simulink model "Satellite_Model_new_seperateSA"  (R2023b)
settings: Solver=ode5  StartTime=0.0  StopTime=10.0  FixedStep=0.1  RelTol=1e-3
undefined symbols (not defined in the file or in its folder): bdf_SA, config_gimbal, epsilon_SA2, f06_SA, gimbal_attach_point, gimbal_cog, gimbal_inertias, gimbal_mass, gimbal_transition_matrix, instrument_attach_point, instrument_inertias, instrument_mass, instrument_transition_matrix, InvDyn, J_B_B, m_B, ObB, ObP1, ObP2, pass, SA, SADM, sig4, unc_freq_SA, uss
libraries: RCTblocks x53, SDTlibV1 x2
(part 1 of 2)
settings Model: Creator=g.iacono  LastModifiedBy=g.iacono

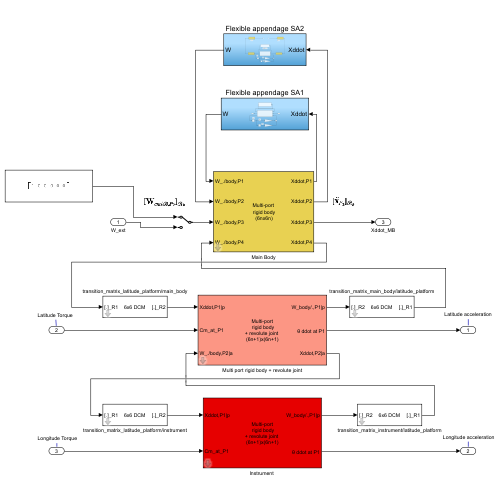
[thumbnail: Simulink's stored preview of the top-level diagram]
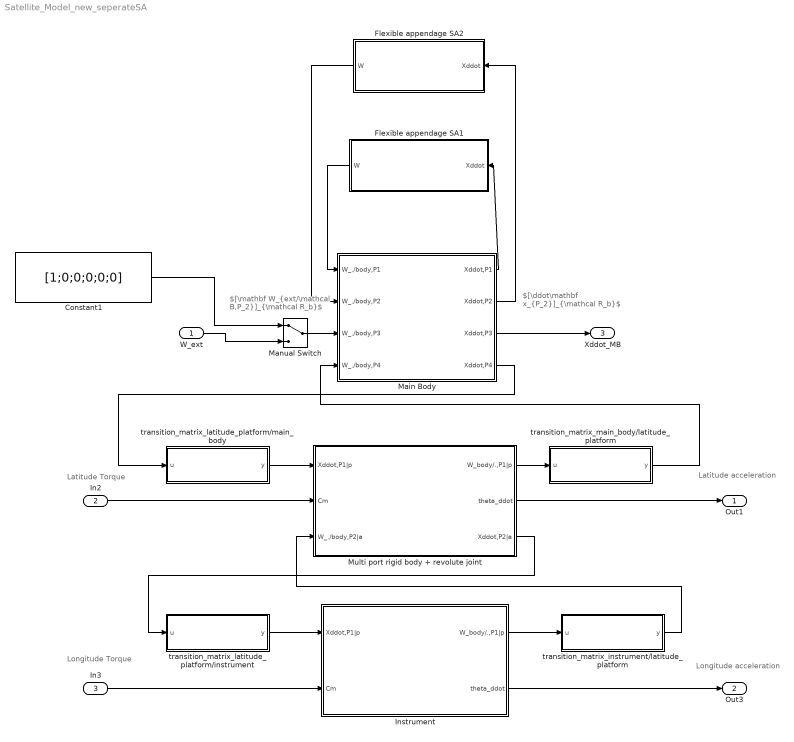
== system Satellite_Model_new_seperateSA ==
  note: Longitude acceleration
  note: Latitude acceleration
  note: $[\ddot\mathbf x_{P_2}]_{\mathcal R_b}$
  note: Longitude Torque
  note: Latitude Torque
  note: $[\mathbf W_{ext/\mathcal B,P_2}]_{\mathcal R_b}$
  W_ext : Inport
  In2 : Inport  Port=2
  In3 : Inport  Port=3
  Constant1 : Constant  Value=[1;0;0;0;0;0]
  Flexible appendage SA1 : Subsystem
  Flexible appendage SA2 : Subsystem
  "Instrument " : Subsystem  mask(Multi-port rigid body with revolute joint (6n+1x6n+1)){m=instrument_mass, Ig=instrument_inertias, OG=instrument_cog-instrument_attach_point, n=1, OP1=[0;0;0], OP2=instrument_attach_point-gimbal_attach_point, OP3=[0;0;0], OP4=[0;0;0], OP5=[0;0;0], ra=[0;1;0], theta=config_gimbal{2}}
      mask prompts: m "Mass (kg)"; Ig "Inertia at G in Ra (kg.m^2)"; OG "OG (3x1 vector in Ra)  (m)"; n "n (number of connection points)"; OP1 "OP1 (3x1 vector in Ra) (m)"; OP2 "OP2 (3x1 vector in Ra) (m)"; OP3 "OP3 (3x1 vector in Ra) (m)"; OP4 "OP4 (3x1 vector in Ra) (m)"; OP5 "OP5 (3x1 vector in Ra) (m)"; ra "ra (joint axis) (3x1 vector)"; theta "Angular configuration (rad)"
      mask help:
      | Computes the (6n+1)x(6n+1) model :
      | - 6x6 transfer from the acceleration twist to the wrench applied by this body to a parent body at port P1 through a revolute joint
      | - the channel # 7 is the transfer:
      |               * from  the  joint torque applied by the input (parent) shaft to the output (body) shaft
      |               * to the relative angular acceleration of the output shaft w.r.t the input shaft.
      | - (n-1) 6x6 transfers from the wrenches applied to this body to the acceleration twists at ports P2,P3,..,
      |
      | Input/Output of port P1 are expressed in the parent frame Rp
      | Input/Output of ports P2,P3,... are expressed in the body frame Ra.
      |
      | O: the body reference point
      | G: the center of mass
      | Pi (i=1:n): the n given connection points or ports (n<6).
      | ra: direction of the revolute joint in the Rp (or Ra)
      | theta: angular configuration of the joint (Ra is obtained from Rp by a rotation of theta around ra).
      |
      | All parameters must be expressed in the body frame Ra.
      | Each parameter can be an uncertain parameter declared with the function ureal (except ra)
      |
      | Rk: if "theta" field is: ureal('NAME',0,'Range',[-pi pi])
      | then, ULINEARIZE will provide a model involving the block named "tan_NAME_div4";
      mask init:
      | MultiPortRigidBodyRev
      mask Help: web('DocMultiportRigidBodyRevolute.html')
      mask TypeOptions n: 1 | 2 | 3 | 4 | 5
      mask DialogControl ParameterGroupVar Prompt: Rigid body parameter
      mask DialogControl port1 Prompt: #1
      mask DialogControl port2 Prompt: #2
      mask DialogControl port3 Prompt: #3
      mask DialogControl port4 Prompt: #4
      mask DialogControl port5 Prompt: #5
      mask DialogControl JointParameters Prompt: Revolute joint parameters
      mask Display:
      | disp('Multi-port\n rigid body\n+ revolute joint \n(6n+1)x(6n+1)')
      | 
      | port_label('input', 1,'Xddot,P1|p')
      | port_label('output',1,'W_body/.,P1|p')
      | port_label('input', 2,'Cm_at_P1')
      | port_label('output',2,'\theta ddot at P1','interpreter','tex')
      | 
      | if n>1
      |     for i=2:n
      |         port_label('input', i+1,['W_./body,P',num2str(i),'|a'])
      |         port_label('output',i+1,['Xddot,P',num2str(i),'|a'])
      |     end
      | end
  Main Body : Subsystem  mask(Multi-port rigid body (6nx6n)){m=m_B, Ig=J_B_B, OG=ObB, n=4, numinv=none, OP1=ObP1, OP2=ObP2, OP3=ObB, OP4=[0;0;0], OP5=[0;0;0]}
      mask prompts: m "Mass (Kg)"; Ig "Inertia (at G, Kg m^2)"; OG "OG (3x1 vector, m)"; n "Number of ports"; numinv "Port to be inverted"; OP1 "OP1 (3x1 vector, m)"; OP2 "OP2 (3x1 vector, m)"; OP3 "OP3 (3x1 vector, m)"; OP4 "OP4 (3x1 vector, m)"; OP5 "OP5 (3x1 vector,m)"
      mask help:
      | 6nx6n dynamic model of a rigid body at n given points (ports) between wrenches applied at the n points (input) and acceleration twists at these points (output).
      |
      | 0: the reference point
      | G: the center of mass
      | Pi (i=1:n): the n given connection points (n<6).
      |
      | All parameters are expressed in the body frame.
      | Each parameter can be an uncertain parameter declared with "ureal"
      |
      | The 6x6 channel associated to one port can be inverted: then the input of this channel is the acceleration twist imposed at this point and the output is the wrench applied by this body.
      mask init:
      | MultiPortRigidBody
      mask Help: web('Docmultiportrigidbody.html')
      mask TypeOptions n: 1 | 2 | 3 | 4 | 5
      mask TypeOptions numinv: none | 1 | 2 | 3 | 4 | 5
      mask DialogControl ParameterGroupVar Prompt: Main parameters
      mask DialogControl port1 Prompt: Port #1
      mask DialogControl port2 Prompt: #2
      mask DialogControl port3 Prompt: #3
      mask DialogControl port4 Prompt: #4
      mask DialogControl port5 Prompt: #5
      mask Display:
      | disp('Multi-port\n rigid body\n (6nx6n)')
      | if n==1,
      |     if numinv-1==1,
      |         port_label('input', 1,'Xddot,P')
      |         port_label('output',1,'W_body/.,P')
      |     else
      |         port_label('input', 1,'W_./body,P')
      |         port_label('output',1,'Xddot,P')
      |     end
      | else
      |     for ii=1:n
      |         if numinv==ii+1,
      |             port_label('output',ii,['W_body/.,P',num2str(ii)])
      |             port_label('input', ii,['Xddot,P',num2str(ii)])
      |         else
      |             port_label('input', ii,['W_./body,P',num2str(ii)])
      |             port_label('output',ii,['Xddot,P',num2str(ii)])
      |         end
      |     end
      | end
  Manual Switch : ManualSwitch
  Multi port rigid body + revolute joint : Subsystem  mask(Multi-port rigid body with revolute joint (6n+1x6n+1)){m=gimbal_mass, Ig=gimbal_inertias, OG=-gimbal_cog+gimbal_attach_point, n=2, OP1=[0;0;0], OP2=-instrument_attach_point+gimbal_attach_point, OP3=[0;0;0], OP4=[0;0;0], OP5=[0;0;0], ra=[1;0;0], theta=config_gimbal{1}}
      mask prompts: m "Mass (kg)"; Ig "Inertia at G in Ra (kg.m^2)"; OG "OG (3x1 vector in Ra)  (m)"; n "n (number of connection points)"; OP1 "OP1 (3x1 vector in Ra) (m)"; OP2 "OP2 (3x1 vector in Ra) (m)"; OP3 "OP3 (3x1 vector in Ra) (m)"; OP4 "OP4 (3x1 vector in Ra) (m)"; OP5 "OP5 (3x1 vector in Ra) (m)"; ra "ra (joint axis) (3x1 vector)"; theta "Angular configuration (rad)"
      mask help:
      | Computes the (6n+1)x(6n+1) model :
      | - 6x6 transfer from the acceleration twist to the wrench applied by this body to a parent body at port P1 through a revolute joint
      | - the channel # 7 is the transfer:
      |               * from  the  joint torque applied by the input (parent) shaft to the output (body) shaft
      |               * to the relative angular acceleration of the output shaft w.r.t the input shaft.
      | - (n-1) 6x6 transfers from the wrenches applied to this body to the acceleration twists at ports P2,P3,..,
      |
      | Input/Output of port P1 are expressed in the parent frame Rp
      | Input/Output of ports P2,P3,... are expressed in the body frame Ra.
      |
      | O: the body reference point
      | G: the center of mass
      | Pi (i=1:n): the n given connection points or ports (n<6).
      | ra: direction of the revolute joint in the Rp (or Ra)
      | theta: angular configuration of the joint (Ra is obtained from Rp by a rotation of theta around ra).
      |
      | All parameters must be expressed in the body frame Ra.
      | Each parameter can be an uncertain parameter declared with the function ureal (except ra)
      |
      | Rk: if "theta" field is: ureal('NAME',0,'Range',[-pi pi])
      | then, ULINEARIZE will provide a model involving the block named "tan_NAME_div4";
      mask init:
      | MultiPortRigidBodyRev
      mask Help: web('DocMultiportRigidBodyRevolute.html')
      mask TypeOptions n: 1 | 2 | 3 | 4 | 5
      mask DialogControl ParameterGroupVar Prompt: Rigid body parameter
      mask DialogControl port1 Prompt: #1
      mask DialogControl port2 Prompt: #2
      mask DialogControl port3 Prompt: #3
      mask DialogControl port4 Prompt: #4
      mask DialogControl port5 Prompt: #5
      mask DialogControl JointParameters Prompt: Revolute joint parameters
      mask Display:
      | disp('Multi-port\n rigid body\n+ revolute joint \n(6n+1)x(6n+1)')
      | 
      | port_label('input', 1,'Xddot,P1|p')
      | port_label('output',1,'W_body/.,P1|p')
      | port_label('input', 2,'Cm_at_P1')
      | port_label('output',2,'\theta ddot at P1','interpreter','tex')
      | 
      | if n>1
      |     for i=2:n
      |         port_label('input', i+1,['W_./body,P',num2str(i),'|a'])
      |         port_label('output',i+1,['Xddot,P',num2str(i),'|a'])
      |     end
      | end
  transition_matrix_instrument/latitude_platform : Subsystem  mask(6x6 Direction cosine matrix (DCM)){rot=instrument_transition_matrix, transp=off}
      mask prompts: rot "3x3 DCM"; transp "Matrix transposed"
      mask help:
      | For 6 d.o.f. body motion (3 translations and 3 rotations), this block Implement the 6x6 rotation matrix (or its transposed) for a given 3x3 DCM.
      |
      | Considering 2 frames R1 and  R2, the DCM between R1 and R2 is defined as the 3x3 matrix where each column is the component vector of each R2 orthogonal unit vector expressed in R1. Thus
      |
      |    [v]_R1 = DCM  * [v]_R2.
      mask init:
      | if transp,
      |     rot=rot';
      | end
      mask Help: web('Doc6dcm.html')
      mask Display:
      | disp('6x6 DCM')
      | if transp
      |     port_label('input', 1, '[.]_R1')
      |     port_label('output', 1, '[.]_R2')
      | else
      |     port_label('input', 1, '[.]_R2')
      |     port_label('output', 1, '[.]_R1')
      | end
  transition_matrix_latitude_platform/instrument : Subsystem  mask(6x6 Direction cosine matrix (DCM)){rot=instrument_transition_matrix, transp=on}
      mask prompts: rot "3x3 DCM"; transp "Matrix transposed"
      mask help:
      | For 6 d.o.f. body motion (3 translations and 3 rotations), this block Implement the 6x6 rotation matrix (or its transposed) for a given 3x3 DCM.
      |
      | Considering 2 frames R1 and  R2, the DCM between R1 and R2 is defined as the 3x3 matrix where each column is the component vector of each R2 orthogonal unit vector expressed in R1. Thus
      |
      |    [v]_R1 = DCM  * [v]_R2.
      mask init:
      | if transp,
      |     rot=rot';
      | end
      mask Help: web('Doc6dcm.html')
      mask Display:
      | disp('6x6 DCM')
      | if transp
      |     port_label('input', 1, '[.]_R1')
      |     port_label('output', 1, '[.]_R2')
      | else
      |     port_label('input', 1, '[.]_R2')
      |     port_label('output', 1, '[.]_R1')
      | end
  transition_matrix_latitude_platform/main_body : Subsystem  mask(6x6 Direction cosine matrix (DCM)){rot=gimbal_transition_matrix, transp=on}
      mask prompts: rot "3x3 DCM"; transp "Matrix transposed"
      mask help:
      | For 6 d.o.f. body motion (3 translations and 3 rotations), this block Implement the 6x6 rotation matrix (or its transposed) for a given 3x3 DCM.
      |
      | Considering 2 frames R1 and  R2, the DCM between R1 and R2 is defined as the 3x3 matrix where each column is the component vector of each R2 orthogonal unit vector expressed in R1. Thus
      |
      |    [v]_R1 = DCM  * [v]_R2.
      mask init:
      | if transp,
      |     rot=rot';
      | end
      mask Help: web('Doc6dcm.html')
      mask Display:
      | disp('6x6 DCM')
      | if transp
      |     port_label('input', 1, '[.]_R1')
      |     port_label('output', 1, '[.]_R2')
      | else
      |     port_label('input', 1, '[.]_R2')
      |     port_label('output', 1, '[.]_R1')
      | end
  transition_matrix_main_body/latitude_platform : Subsystem  mask(6x6 Direction cosine matrix (DCM)){rot=gimbal_transition_matrix, transp=off}
      mask prompts: rot "3x3 DCM"; transp "Matrix transposed"
      mask help:
      | For 6 d.o.f. body motion (3 translations and 3 rotations), this block Implement the 6x6 rotation matrix (or its transposed) for a given 3x3 DCM.
      |
      | Considering 2 frames R1 and  R2, the DCM between R1 and R2 is defined as the 3x3 matrix where each column is the component vector of each R2 orthogonal unit vector expressed in R1. Thus
      |
      |    [v]_R1 = DCM  * [v]_R2.
      mask init:
      | if transp,
      |     rot=rot';
      | end
      mask Help: web('Doc6dcm.html')
      mask Display:
      | disp('6x6 DCM')
      | if transp
      |     port_label('input', 1, '[.]_R1')
      |     port_label('output', 1, '[.]_R2')
      | else
      |     port_label('input', 1, '[.]_R2')
      |     port_label('output', 1, '[.]_R1')
      | end
  Out1 : Outport  VectorParamsAs1DForOutWhenUnconnected=off
  Out3 : Outport  Port=2  VectorParamsAs1DForOutWhenUnconnected=off
  Xddot_MB : Outport  Port=3
  wires:
  Multi port rigid body + revolute joint/3(Xddot,P2|a) -> transition_matrix_latitude_platform/instrument/1(u)
  Main Body/3(Xddot,P3) -> Xddot_MB/1
  W_ext/1 -> Manual Switch/2
  "Instrument "/2(theta_ddot) -> Out3/1
  In3/1 -> "Instrument "/2(Cm)
  transition_matrix_latitude_platform/instrument/1(y) -> "Instrument "/1(Xddot,P1|p)
  Multi port rigid body + revolute joint/2(theta_ddot) -> Out1/1
  transition_matrix_latitude_platform/main_body/1(y) -> Multi port rigid body + revolute joint/1(Xddot,P1|p)
  Multi port rigid body + revolute joint/1(W_body/.,P1|p) -> transition_matrix_main_body/latitude_platform/1(u)
  "Instrument "/1(W_body/.,P1|p) -> transition_matrix_instrument/latitude_platform/1(u)
  Flexible appendage SA1/1(W) -> Main Body/1(W_./body,P1)
  transition_matrix_main_body/latitude_platform/1(y) -> Main Body/4(W_./body,P4)
  transition_matrix_instrument/latitude_platform/1(y) -> Multi port rigid body + revolute joint/3(W_./body,P2|a)
  In2/1 -> Multi port rigid body + revolute joint/2(Cm)
  Main Body/1(Xddot,P1) -> Flexible appendage SA1/1(Xddot)
  Main Body/4(Xddot,P4) -> transition_matrix_latitude_platform/main_body/1(u)
  Main Body/2(Xddot,P2) -> Flexible appendage SA2/1(Xddot)
  Flexible appendage SA2/1(W) -> Main Body/2(W_./body,P2)
  Manual Switch/1 -> Main Body/3(W_./body,P3)
  Constant1/1 -> Manual Switch/1

== system Satellite_Model_new_seperateSA/Flexible appendage SA1 ==
  note: $\dot{\delta\theta}_1$
  note: $\delta\theta_1$
  note: $\ddot{\delta\theta}_1$
  Xddot : Inport
  Gain1 : Gain  Gain=SADM.damping
  Gain4 : Gain  Gain=SADM.Stiffness
  Integrator1 : Integrator
  Integrator4 : Integrator
  SADM1 : SDTlibV1/6 dof mechanisms/Revolute joint + configuration  ra=[1;0;0]  Jr=1e-9  theta=theta_SA
      settings: SourceProductName=SDTlib
  Solar Array 1 : Subsystem  mask(NINOP Model of a Nastran body){fbdf=bdf_SA, ff06=f06_SA, P_gp=SA.pointP, C_gp=[], nf=SA.n_modes, Xi=SA.damping_ratio, uw_var=unc_freq_SA, Nflex_w=SA.n_unc, uls_var=SA.MPCunc, Nflex_LP=SA.n_MPCunc, uev_var=0, Nflex_EV=0}
      mask prompts: fbdf "Name of the .bdf file (without extension)"; ff06 "Name of the .f06 file (without extension)"; P_gp "Node number corresponding to the point P (connection with parent body)"; C_gp "Node numbers corresponding to the points C (connections with child bodies)"; nf "Number of modes to be considered"; Xi "Common damping ratio"; uw_var "uncertainties (%)"; Nflex_w "number of flexible modes (integer)"; uls_var "uncertainties (%)"; Nflex_LP "number of flexible modes (integer)"; uev_var "uncertainties (%)"; Nflex_EV "number of flexible modes (integer)"
      mask help:
      | NINOP 6(n+1)x6(n+1) model of a flexible body at points C (connection point with the child  bodies) and point P (connection point with a parent body).
      | * 6nx6n transfer between the wrench applied to this body at the child points C  and accelaretion twist at these points
      | * 6x6 transfer between the acceleration twist at the "parent" point P  and the wrench applied by this body at this point
      | The model is expressed In the (inherit) body frame.
      |
      | Model is built from  the data provided by Patran/Nastran analysis output files.
      | Uncertainties can be added to the main parameters
      mask init:
      | n = length(C_gp);
      | NastranBodyNPort
      mask Help: web('DocNPortNastranBody.html')
      mask DialogControl Container2 Prompt: Main parameters
      mask DialogControl Container6 Prompt: Parametric uncertainties:
      mask DialogControl Container8 Prompt: Frequencies
      mask DialogControl Control18 Prompt: A common relative uncertainty (%) on the first flexible mode frequencies can be added (uncertainties can be changed later)
      mask DialogControl Control3 Prompt: The uncertain frequency is named: 'w_name_i' where:
      mask DialogControl Control4 Prompt: * 'name' is the current block name (reduced to its alphanumeric characters).
      mask DialogControl Control17 Prompt: * 'i' is the flexible mode number (increasing frequency order)
      mask DialogControl Container9 Prompt: Modal participation factors
      mask DialogControl Control20 Prompt: A common relative uncertainty (%) on the modal participation factors of the first flexible modes can be added (uncertainties can be changed later)
      mask DialogControl Control6 Prompt: The uncertain modal participation factor is named: 'LP_name_iXX' where:
      mask DialogControl Control7 Prompt: *  'name' is the current block name (reduced to its alphanumeric characters),
      mask DialogControl Control8 Prompt: * 'i' is the flexible mode number (increasing frequency order),
      mask DialogControl Control9 Prompt: * 'XX' = 'Tx', 'Ty', 'Tz', 'Rx', 'Ry', 'Rz'.
      mask DialogControl Container10 Prompt: Modal shapes
      mask DialogControl Control21 Prompt: A common relative uncertainty (%) on each eigen vector components at points C for the first flexible modes can be added (uncertainties can be changed later)
      mask DialogControl Control16 Prompt: WARNING: can generate very long process time !!
      mask DialogControl Control11 Prompt: The uncertain component is named: "EV_name_Cj_iXX' where:
      mask DialogControl Control12 Prompt: * 'name' is the current block name (reduced to its alphanumeric characters).
      mask DialogControl Control13 Prompt: * 'j' is the point C number,
      mask DialogControl Control14 Prompt: * 'i' is the flexible mode number (increasing frequency order),
      mask DialogControl Control15 Prompt: * 'XX' = 'Tx', 'Ty', 'Tz', 'Rx', 'Ry', 'Rz'.
      mask Display:
      | disp('NINOP\n Nastran body\n (6(n+1)x6(n+1))')
      | 
      | 
      | for ii=1:n
      |         port_label('input', ii,['W_./body,C',num2str(ii)])
      |         port_label('output',ii,['Xddot,C',num2str(ii)])
      | end
      | 
      | port_label('input', n+1,'Xddot,P')
      | port_label('output',n+1,'Wbody/.,P')
  Sum4 : Sum  Inputs=++|
  W : Outport
  wires:
  SADM1/2 -> W/1
  Xddot/1 -> SADM1/2
  Sum4/1 -> SADM1/3
  Integrator1/1 -> Integrator4/1, Gain1/1
  Gain1/1 -> Sum4/1
  Integrator4/1 -> Gain4/1
  Gain4/1 -> Sum4/2
  SADM1/3 -> Integrator1/1
  SADM1/1 -> Solar Array 1/1(Xddot,P)
  Solar Array 1/1(W_body/.,P) -> SADM1/1

== system Satellite_Model_new_seperateSA/Flexible appendage SA2 ==
  note: $-[\mathbf M^{\mathcal A_2}_{P_2}]_{\mathcal R_{a_2}}(\mathrm s)$
  note: $\mathbf P_{a_2(0)/b}$
  note: $\mathbf P_{a_2(0)/b}^T$
  note: $\ddot{\delta\theta}_2$
  note: $\delta\theta_2$
  note: $\dot{\delta\theta}_2$
  Xddot : Inport
  6x6 DCM1 : Subsystem  mask(6x6 Direction cosine matrix (DCM)){rot=[-1 0 0;0 -1 0;0 0 1], transp=off}
      mask prompts: rot "3x3 DCM"; transp "Matrix transposed"
      mask help:
      | For 6 d.o.f. body motion (3 translations and 3 rotations), this block Implement the 6x6 rotation matrix (or its transposed) for a given 3x3 DCM.
      |
      | Considering 2 frames R1 and  R2, the DCM between R1 and R2 is defined as the 3x3 matrix where each column is the component vector of each R2 orthogonal unit vector expressed in R1. Thus
      |
      |    [v]_R1 = DCM  * [v]_R2.
      mask init:
      | if transp,
      |     rot=rot';
      | end
      mask Help: web('Doc6dcm.html')
      mask Display:
      | disp('6x6 DCM')
      | if transp
      |     port_label('input', 1, '[.]_R1')
      |     port_label('output', 1, '[.]_R2')
      | else
      |     port_label('input', 1, '[.]_R2')
      |     port_label('output', 1, '[.]_R1')
      | end
  6x6 DCM2 : Subsystem  mask(6x6 Direction cosine matrix (DCM)){rot=[-1 0 0;0 -1 0;0 0 1], transp=on}
      mask prompts: rot "3x3 DCM"; transp "Matrix transposed"
      mask help:
      | For 6 d.o.f. body motion (3 translations and 3 rotations), this block Implement the 6x6 rotation matrix (or its transposed) for a given 3x3 DCM.
      |
      | Considering 2 frames R1 and  R2, the DCM between R1 and R2 is defined as the 3x3 matrix where each column is the component vector of each R2 orthogonal unit vector expressed in R1. Thus
      |
      |    [v]_R1 = DCM  * [v]_R2.
      mask init:
      | if transp,
      |     rot=rot';
      | end
      mask Help: web('Doc6dcm.html')
      mask Display:
      | disp('6x6 DCM')
      | if transp
      |     port_label('input', 1, '[.]_R1')
      |     port_label('output', 1, '[.]_R2')
      | else
      |     port_label('input', 1, '[.]_R2')
      |     port_label('output', 1, '[.]_R1')
      | end
  6x6 v-u_rotation2 : Subsystem  mask(6x6 rotation matrix (around a given axis)){ra=[-1;0;0], theta=epsilon_SA2, transp=on}
      mask prompts: ra "Rotation axis (3x1 vector)"; theta "Angle (rad)"; transp "Matrix transposed"
      mask help:
      | For 6 d.o.f. body motion (3 translations and 3 rotations), this block Implement the 6x6 rotation matrix (or its transposed) for a given angle around a given axis.
      |
      | Angle  (rad) can be an uncertain parameter declared with "ureal" with mode 'Range'
      | Ex: ureal('NAME',0,'Range',[-pi pi])
      | Then, ULINEARIZE will provide a model involving the block named "tan_NAME_div4".
      mask init:
      | vUrotation3x3
      mask Help: web('Doc6vurotation.html')
      mask Display:
      | disp('v-rot\n6x6')
      | if transp
      |     port_label('input', 1, '[.]_R1')
      |     port_label('output', 1, '[.]_R2')
      | else
      |     port_label('input', 1, '[.]_R2')
      |     port_label('output', 1, '[.]_R1')
      | end
  6x6 v-u_rotation3 : Subsystem  mask(6x6 rotation matrix (around a given axis)){ra=[-1;0;0], theta=epsilon_SA2, transp=off}
      mask prompts: ra "Rotation axis (3x1 vector)"; theta "Angle (rad)"; transp "Matrix transposed"
      mask help:
      | For 6 d.o.f. body motion (3 translations and 3 rotations), this block Implement the 6x6 rotation matrix (or its transposed) for a given angle around a given axis.
      |
      | Angle  (rad) can be an uncertain parameter declared with "ureal" with mode 'Range'
      | Ex: ureal('NAME',0,'Range',[-pi pi])
      | Then, ULINEARIZE will provide a model involving the block named "tan_NAME_div4".
      mask init:
      | vUrotation3x3
      mask Help: web('Doc6vurotation.html')
      mask Display:
      | disp('v-rot\n6x6')
      | if transp
      |     port_label('input', 1, '[.]_R1')
      |     port_label('output', 1, '[.]_R2')
      | else
      |     port_label('input', 1, '[.]_R2')
      |     port_label('output', 1, '[.]_R1')
      | end
  Gain2 : Gain  Gain=SADM.damping
  Gain3 : Gain  Gain=SADM.Stiffness
  Integrator2 : Integrator
  Integrator3 : Integrator
  SADM2 : SDTlibV1/6 dof mechanisms/Revolute joint + configuration  ra=[-1;0;0]  Jr=1e-9  theta=theta_SA
      settings: SourceProductName=SDTlib
  Solar Array 2 : Subsystem  mask(NINOP Model of a Nastran body){fbdf=bdf_SA, ff06=f06_SA, P_gp=SA.pointP, C_gp=[], nf=SA.n_modes, Xi=SA.damping_ratio, uw_var=unc_freq_SA, Nflex_w=SA.n_unc, uls_var=SA.MPCunc, Nflex_LP=SA.n_MPCunc, uev_var=0, Nflex_EV=0}
      mask prompts: fbdf "Name of the .bdf file (without extension)"; ff06 "Name of the .f06 file (without extension)"; P_gp "Node number corresponding to the point P (connection with parent body)"; C_gp "Node numbers corresponding to the points C (connections with child bodies)"; nf "Number of modes to be considered"; Xi "Common damping ratio"; uw_var "uncertainties (%)"; Nflex_w "number of flexible modes (integer)"; uls_var "uncertainties (%)"; Nflex_LP "number of flexible modes (integer)"; uev_var "uncertainties (%)"; Nflex_EV "number of flexible modes (integer)"
      mask help:
      | NINOP 6(n+1)x6(n+1) model of a flexible body at points C (connection point with the child  bodies) and point P (connection point with a parent body).
      | * 6nx6n transfer between the wrench applied to this body at the child points C  and accelaretion twist at these points
      | * 6x6 transfer between the acceleration twist at the "parent" point P  and the wrench applied by this body at this point
      | The model is expressed In the (inherit) body frame.
      |
      | Model is built from  the data provided by Patran/Nastran analysis output files.
      | Uncertainties can be added to the main parameters
      mask init:
      | n = length(C_gp);
      | NastranBodyNPort
      mask Help: web('DocNPortNastranBody.html')
      mask DialogControl Container2 Prompt: Main parameters
      mask DialogControl Container6 Prompt: Parametric uncertainties:
      mask DialogControl Container8 Prompt: Frequencies
      mask DialogControl Control18 Prompt: A common relative uncertainty (%) on the first flexible mode frequencies can be added (uncertainties can be changed later)
      mask DialogControl Control3 Prompt: The uncertain frequency is named: 'w_name_i' where:
      mask DialogControl Control4 Prompt: * 'name' is the current block name (reduced to its alphanumeric characters).
      mask DialogControl Control17 Prompt: * 'i' is the flexible mode number (increasing frequency order)
      mask DialogControl Container9 Prompt: Modal participation factors
      mask DialogControl Control20 Prompt: A common relative uncertainty (%) on the modal participation factors of the first flexible modes can be added (uncertainties can be changed later)
      mask DialogControl Control6 Prompt: The uncertain modal participation factor is named: 'LP_name_iXX' where:
      mask DialogControl Control7 Prompt: *  'name' is the current block name (reduced to its alphanumeric characters),
      mask DialogControl Control8 Prompt: * 'i' is the flexible mode number (increasing frequency order),
      mask DialogControl Control9 Prompt: * 'XX' = 'Tx', 'Ty', 'Tz', 'Rx', 'Ry', 'Rz'.
      mask DialogControl Container10 Prompt: Modal shapes
      mask DialogControl Control21 Prompt: A common relative uncertainty (%) on each eigen vector components at points C for the first flexible modes can be added (uncertainties can be changed later)
      mask DialogControl Control16 Prompt: WARNING: can generate very long process time !!
      mask DialogControl Control11 Prompt: The uncertain component is named: "EV_name_Cj_iXX' where:
      mask DialogControl Control12 Prompt: * 'name' is the current block name (reduced to its alphanumeric characters).
      mask DialogControl Control13 Prompt: * 'j' is the point C number,
      mask DialogControl Control14 Prompt: * 'i' is the flexible mode number (increasing frequency order),
      mask DialogControl Control15 Prompt: * 'XX' = 'Tx', 'Ty', 'Tz', 'Rx', 'Ry', 'Rz'.
      mask Display:
      | disp('NINOP\n Nastran body\n (6(n+1)x6(n+1))')
      | 
      | 
      | for ii=1:n
      |         port_label('input', ii,['W_./body,C',num2str(ii)])
      |         port_label('output',ii,['Xddot,C',num2str(ii)])
      | end
      | 
      | port_label('input', n+1,'Xddot,P')
      | port_label('output',n+1,'Wbody/.,P')
  Sum3 : Sum  Inputs=++|
  W : Outport
  wires:
  SADM2/1 -> Solar Array 2/1(Xddot,P)
  Xddot/1 -> 6x6 DCM2/1(u)
  6x6 DCM1/1(y) -> W/1
  6x6 DCM2/1(y) -> 6x6 v-u_rotation2/1(u)
  Solar Array 2/1(W_body/.,P) -> SADM2/1
  SADM2/2 -> 6x6 v-u_rotation3/1(u)
  6x6 v-u_rotation2/1(y) -> SADM2/2
  6x6 v-u_rotation3/1(y) -> 6x6 DCM1/1(u)
  SADM2/3 -> Integrator2/1
  Gain3/1 -> Sum3/2
  Integrator3/1 -> Gain3/1
  Gain2/1 -> Sum3/1
  Integrator2/1 -> Integrator3/1, Gain2/1
  Sum3/1 -> SADM2/3

== system Satellite_Model_new_seperateSA/Instrument  ==
  Xddot,P1|p : Inport
  Cm : Inport  Port=2
  Multi port rigid body : Subsystem  mask(Multi-port rigid body (6nx6n)){m=instrument_mass, Ig=[1 0 0;0 0.0005 0;0 0 0.001], OG=instrument_cog-instrument_attach_point, n=1, numinv=1, OP1=[0;0;0], OP2=instrument_attach_point-gimbal_attach_point, OP3=[0;0;0], OP4=[0;0;0], OP5=[0;0;0]}
      mask prompts: m "Mass (Kg)"; Ig "Inertia (at G, Kg m^2)"; OG "OG (3x1 vector, m)"; n "Number of ports"; numinv "Port to be inverted"; OP1 "OP1 (3x1 vector, m)"; OP2 "OP2 (3x1 vector, m)"; OP3 "OP3 (3x1 vector, m)"; OP4 "OP4 (3x1 vector, m)"; OP5 "OP5 (3x1 vector,m)"
      mask help:
      | 6nx6n inverse dynamic model between:
      |    *  wrenches applied to this body at the given n points,
      |    * acceleration twiists at he n given points.
      |
      | The 6x6 channel asociated to a single given point can be inverted
      mask init:
      | MultiPortRigidBody
      mask Help: web('Docmultiportrigidbody.html')
      mask TypeOptions n: 1 | 2 | 3 | 4 | 5
      mask TypeOptions numinv: none | 1 | 2 | 3 | 4 | 5
      mask DialogControl Control1 Prompt: Inverse Dynamic model of a rigid body at n given points (ports):
      mask DialogControl Control2 Prompt: 6nx6n transfer between wrenches applied at the n points and accelaretion twists at these points
      mask DialogControl Control3 Prompt: 0: the reference point
      mask DialogControl Control4 Prompt: G: the center of mass
      mask DialogControl Control5 Prompt: Pi (i=1:n): the n given connection points (n<6).
      mask DialogControl Control6 Prompt: All parameters are expressed in the body frame.
      mask DialogControl Control7 Prompt: Each parameter can be an uncertain parameter declared with "ureal"
      mask DialogControl Control8 Prompt: The 6x6 channel associated to one port can be inverted: then the input of this channel is the acceleration twist imposed at this point and the output is the wrench applied by this body.
      mask DialogControl ParameterGroupVar Prompt: Main parameters
      mask DialogControl port1 Prompt: Port #1
      mask DialogControl port2 Prompt: #2
      mask DialogControl port3 Prompt: #3
      mask DialogControl port4 Prompt: #4
      mask DialogControl port5 Prompt: #5
      mask Display:
      | disp('Multi-port\n rigid body\n (6nx6n)')
      | if n==1,
      |     if numinv-1==1,
      |         port_label('input', 1,'Xddot,P')
      |         port_label('output',1,'W_body/.,P')
      |     else
      |         port_label('input', 1,'W_./body,P')
      |         port_label('output',1,'Xddot,P')
      |     end
      | else
      |     for ii=1:n
      |         if numinv==ii+1,
      |             port_label('output',ii,['W_body/.,P',num2str(ii)])
      |             port_label('input', ii,['Xddot,P',num2str(ii)])
      |         else
      |             port_label('input', ii,['W_./body,P',num2str(ii)])
      |             port_label('output',ii,['Xddot,P',num2str(ii)])
      |         end
      |     end
      | end
  Revolute joint + configuration : Subsystem  mask(Revolute joint){ra=[0;1;0], Jr=0.0005, theta=config_gimbal{2}}
      mask prompts: ra "Direction of the joint in the load frame (3x1 vector)"; Jr "Rotor inertia (kg.m^2)"; theta "Angular configuration (rad)"
      mask help:
      | This block implement the TITOP model of of a revolute joint.
      | The last channel is the transfer between the torque applied inside the joint by the input shaft to the output shaft and the relative angular acceleration of the output shaft w.r.t the input shaft.
      |
      | Angular configuration can be a vayring parameter: Ex:
      | ureal('NAME',0,'Range',[-pi pi])
      |
      | Then, ULINEARIZE will provide a model involving the block named "tan_NAME_div4";
      mask init:
      | pass=ra2DCMi(ra);
      mask Help: web('DocRevoluteJoint_configuration.html')
      mask Display:
      | disp('Revolute joint\nTITOP model\n+ angle configuration')
      | port_label('input', 1, 'W_./r|a')
      | port_label('output', 1, 'Xddot_out|a')
      | port_label('input', 2, 'Xddot_in|p')
      | port_label('output', 2, 'W_r/.|p')
      | port_label('input', 3, 'Cm')
      | port_label('output', 3, '\theta ddot','interpreter','tex')
  W_body/.,P1|p : Outport  VectorParamsAs1DForOutWhenUnconnected=off
  theta_ddot : Outport  Port=2  VectorParamsAs1DForOutWhenUnconnected=off
  wires:
  Revolute joint + configuration/1(Xddot_out|a) -> Multi port rigid body/1(Xddot,P1)
  Multi port rigid body/1(W_body/.,P1) -> Revolute joint + configuration/1(W_./r|a)
  Xddot,P1|p/1 -> Revolute joint + configuration/2(Xddot_in|p)
  Cm/1 -> Revolute joint + configuration/3(Cm)
  Revolute joint + configuration/2(W_r/.|p) -> W_body/.,P1|p/1
  Revolute joint + configuration/3(Theta_ddot) -> theta_ddot/1

== system Satellite_Model_new_seperateSA/Main Body ==
  W_./body,P1 : Inport  PortDimensions=6
  W_./body,P2 : Inport  Port=2  PortDimensions=6
  W_./body,P3 : Inport  Port=3  PortDimensions=6
  W_./body,P4 : Inport  Port=4  PortDimensions=6
  Demux : Demux  Outputs=[6 6 6 6]
  Gain : RCTblocks/Uncertain State Space  Tag=USS  USystem=uss(InvDyn)  UValue=[]  X0=[]  uX0=[]
  Mux : Mux  Inputs=[6 6 6 6]
  Xddot,P1 : Outport
  Xddot,P2 : Outport  Port=2
  Xddot,P3 : Outport  Port=3
  Xddot,P4 : Outport  Port=4
  wires:
  Mux/1 -> Gain/1
  Gain/1 -> Demux/1
  W_./body,P1/1 -> Mux/1
  Demux/1 -> Xddot,P1/1
  W_./body,P2/1 -> Mux/2
  Demux/2 -> Xddot,P2/1
  W_./body,P3/1 -> Mux/3
  Demux/3 -> Xddot,P3/1
  W_./body,P4/1 -> Mux/4
  Demux/4 -> Xddot,P4/1

== system Satellite_Model_new_seperateSA/Multi port rigid body + revolute joint ==
  Xddot,P1|p : Inport
  Cm : Inport  Port=2
  W_./body,P2|a : Inport  Port=3
  Multi port rigid body : Subsystem  mask(Multi-port rigid body (6nx6n)){m=gimbal_mass, Ig=[-3.1995 0 0;0 4 0;0 0 0.001], OG=-gimbal_cog+gimbal_attach_point, n=2, numinv=1, OP1=[0;0;0], OP2=-instrument_attach_point+gimbal_attach_point, OP3=[0;0;0], OP4=[0;0;0], OP5=[0;0;0]}
      mask prompts: m "Mass (Kg)"; Ig "Inertia (at G, Kg m^2)"; OG "OG (3x1 vector, m)"; n "Number of ports"; numinv "Port to be inverted"; OP1 "OP1 (3x1 vector, m)"; OP2 "OP2 (3x1 vector, m)"; OP3 "OP3 (3x1 vector, m)"; OP4 "OP4 (3x1 vector, m)"; OP5 "OP5 (3x1 vector,m)"
      mask help:
      | 6nx6n inverse dynamic model between:
      |    *  wrenches applied to this body at the given n points,
      |    * acceleration twiists at he n given points.
      |
      | The 6x6 channel asociated to a single given point can be inverted
      mask init:
      | MultiPortRigidBody
      mask Help: web('Docmultiportrigidbody.html')
      mask TypeOptions n: 1 | 2 | 3 | 4 | 5
      mask TypeOptions numinv: none | 1 | 2 | 3 | 4 | 5
      mask DialogControl Control1 Prompt: Inverse Dynamic model of a rigid body at n given points (ports):
      mask DialogControl Control2 Prompt: 6nx6n transfer between wrenches applied at the n points and accelaretion twists at these points
      mask DialogControl Control3 Prompt: 0: the reference point
      mask DialogControl Control4 Prompt: G: the center of mass
      mask DialogControl Control5 Prompt: Pi (i=1:n): the n given connection points (n<6).
      mask DialogControl Control6 Prompt: All parameters are expressed in the body frame.
      mask DialogControl Control7 Prompt: Each parameter can be an uncertain parameter declared with "ureal"
      mask DialogControl Control8 Prompt: The 6x6 channel associated to one port can be inverted: then the input of this channel is the acceleration twist imposed at this point and the output is the wrench applied by this body.
      mask DialogControl ParameterGroupVar Prompt: Main parameters
      mask DialogControl port1 Prompt: Port #1
      mask DialogControl port2 Prompt: #2
      mask DialogControl port3 Prompt: #3
      mask DialogControl port4 Prompt: #4
      mask DialogControl port5 Prompt: #5
      mask Display:
      | disp('Multi-port\n rigid body\n (6nx6n)')
      | if n==1,
      |     if numinv-1==1,
      |         port_label('input', 1,'Xddot,P')
      |         port_label('output',1,'W_body/.,P')
      |     else
      |         port_label('input', 1,'W_./body,P')
      |         port_label('output',1,'Xddot,P')
      |     end
      | else
      |     for ii=1:n
      |         if numinv==ii+1,
      |             port_label('output',ii,['W_body/.,P',num2str(ii)])
      |             port_label('input', ii,['Xddot,P',num2str(ii)])
      |         else
      |             port_label('input', ii,['W_./body,P',num2str(ii)])
      |             port_label('output',ii,['Xddot,P',num2str(ii)])
      |         end
      |     end
      | end
  Revolute joint + configuration : Subsystem  mask(Revolute joint){ra=[1;0;0], Jr=3.2005, theta=config_gimbal{1}}
      mask prompts: ra "Direction of the joint in the load frame (3x1 vector)"; Jr "Rotor inertia (kg.m^2)"; theta "Angular configuration (rad)"
      mask help:
      | This block implement the TITOP model of of a revolute joint.
      | The last channel is the transfer between the torque applied inside the joint by the input shaft to the output shaft and the relative angular acceleration of the output shaft w.r.t the input shaft.
      |
      | Angular configuration can be a vayring parameter: Ex:
      | ureal('NAME',0,'Range',[-pi pi])
      |
      | Then, ULINEARIZE will provide a model involving the block named "tan_NAME_div4";
      mask init:
      | pass=ra2DCMi(ra);
      mask Help: web('DocRevoluteJoint_configuration.html')
      mask Display:
      | disp('Revolute joint\nTITOP model\n+ angle configuration')
      | port_label('input', 1, 'W_./r|a')
      | port_label('output', 1, 'Xddot_out|a')
      | port_label('input', 2, 'Xddot_in|p')
      | port_label('output', 2, 'W_r/.|p')
      | port_label('input', 3, 'Cm')
      | port_label('output', 3, '\theta ddot','interpreter','tex')
  W_body/.,P1|p : Outport  VectorParamsAs1DForOutWhenUnconnected=off
  theta_ddot : Outport  Port=2  VectorParamsAs1DForOutWhenUnconnected=off
  Xddot,P2|a : Outport  Port=3
  wires:
  Revolute joint + configuration/1(Xddot_out|a) -> Multi port rigid body/1(Xddot,P1)
  Multi port rigid body/1(W_body/.,P1) -> Revolute joint + configuration/1(W_./r|a)
  Xddot,P1|p/1 -> Revolute joint + configuration/2(Xddot_in|p)
  Cm/1 -> Revolute joint + configuration/3(Cm)
  Revolute joint + configuration/2(W_r/.|p) -> W_body/.,P1|p/1
  Revolute joint + configuration/3(Theta_ddot) -> theta_ddot/1
  W_./body,P2|a/1 -> Multi port rigid body/2(W_./body,P2)
  Multi port rigid body/2(Xddot,P2) -> Xddot,P2|a/1

== system Satellite_Model_new_seperateSA/transition_matrix_instrument//latitude_platform ==
  u : Inport  PortDimensions=6
  Demux : Demux  Outputs=[3 3]
  Mux : Mux  Inputs=[3 3]
  rotation : Gain  Gain=rot  Multiplication=Matrix(K*u) (u vector)
  translation : Gain  Gain=rot  Multiplication=Matrix(K*u) (u vector)
  y : Outport  VectorParamsAs1DForOutWhenUnconnected=off
  wires:
  rotation/1 -> Mux/2
  translation/1 -> Mux/1
  Demux/1 -> translation/1
  u/1 -> Demux/1
  Mux/1 -> y/1
  Demux/2 -> rotation/1

== system Satellite_Model_new_seperateSA/transition_matrix_latitude_platform//instrument ==
  u : Inport  PortDimensions=6
  Demux : Demux  Outputs=[3 3]
  Mux : Mux  Inputs=[3 3]
  rotation : Gain  Gain=rot  Multiplication=Matrix(K*u) (u vector)
  translation : Gain  Gain=rot  Multiplication=Matrix(K*u) (u vector)
  y : Outport  VectorParamsAs1DForOutWhenUnconnected=off
  wires:
  Demux/2 -> rotation/1
  Mux/1 -> y/1
  u/1 -> Demux/1
  Demux/1 -> translation/1
  translation/1 -> Mux/1
  rotation/1 -> Mux/2

== system Satellite_Model_new_seperateSA/transition_matrix_latitude_platform//main_body ==
  u : Inport  PortDimensions=6
  Demux : Demux  Outputs=[3 3]
  Mux : Mux  Inputs=[3 3]
  rotation : Gain  Gain=rot  Multiplication=Matrix(K*u) (u vector)
  translation : Gain  Gain=rot  Multiplication=Matrix(K*u) (u vector)
  y : Outport  VectorParamsAs1DForOutWhenUnconnected=off
  wires:
  rotation/1 -> Mux/2
  translation/1 -> Mux/1
  Demux/1 -> translation/1
  u/1 -> Demux/1
  Mux/1 -> y/1
  Demux/2 -> rotation/1

== system Satellite_Model_new_seperateSA/transition_matrix_main_body//latitude_platform ==
  u : Inport  PortDimensions=6
  Demux : Demux  Outputs=[3 3]
  Mux : Mux  Inputs=[3 3]
  rotation : Gain  Gain=rot  Multiplication=Matrix(K*u) (u vector)
  translation : Gain  Gain=rot  Multiplication=Matrix(K*u) (u vector)
  y : Outport  VectorParamsAs1DForOutWhenUnconnected=off
  wires:
  rotation/1 -> Mux/2
  translation/1 -> Mux/1
  Demux/1 -> translation/1
  u/1 -> Demux/1
  Mux/1 -> y/1
  Demux/2 -> rotation/1

== system Satellite_Model_new_seperateSA/Flexible appendage SA1/Solar Array 1 ==
  Xddot,P : Inport  PortDimensions=6
  Demux : Demux  Outputs=[6]
  Gain : RCTblocks/Uncertain State Space  Tag=USS  USystem=Mdyn  UValue=[]  X0=[]  uX0=[]
  Mux : Mux  Inputs=[6]
  W_body/.,P : Outport
  wires:
  Demux/1 -> W_body/.,P/1
  Xddot,P/1 -> Mux/1
  Gain/1 -> Demux/1
  Mux/1 -> Gain/1

== system Satellite_Model_new_seperateSA/Flexible appendage SA2/6x6 DCM1 ==
  u : Inport  PortDimensions=6
  Demux : Demux  Outputs=[3 3]
  Mux : Mux  Inputs=[3 3]
  rotation : Gain  Gain=rot  Multiplication=Matrix(K*u) (u vector)
  translation : Gain  Gain=rot  Multiplication=Matrix(K*u) (u vector)
  y : Outport  VectorParamsAs1DForOutWhenUnconnected=off
  wires:
  rotation/1 -> Mux/2
  translation/1 -> Mux/1
  Demux/1 -> translation/1
  u/1 -> Demux/1
  Mux/1 -> y/1
  Demux/2 -> rotation/1

== system Satellite_Model_new_seperateSA/Flexible appendage SA2/6x6 DCM2 ==
  u : Inport  PortDimensions=6
  Demux : Demux  Outputs=[3 3]
  Mux : Mux  Inputs=[3 3]
  rotation : Gain  Gain=rot  Multiplication=Matrix(K*u) (u vector)
  translation : Gain  Gain=rot  Multiplication=Matrix(K*u) (u vector)
  y : Outport  VectorParamsAs1DForOutWhenUnconnected=off
  wires:
  rotation/1 -> Mux/2
  translation/1 -> Mux/1
  Demux/1 -> translation/1
  u/1 -> Demux/1
  Mux/1 -> y/1
  Demux/2 -> rotation/1

== system Satellite_Model_new_seperateSA/Flexible appendage SA2/6x6 v-u_rotation2 ==
  u : Inport  PortDimensions=6
  Demux : Demux  Outputs=[3 3]
  Mux : Mux  Inputs=[3 3]
  Subsystem : Subsystem
  Subsystem1 : Subsystem
  y : Outport  VectorParamsAs1DForOutWhenUnconnected=off
  wires:
  Subsystem1/1(Out1) -> Mux/2
  Subsystem/1(Out1) -> Mux/1
  Demux/2 -> Subsystem1/1(In1)
  Demux/1 -> Subsystem/1(In1)
  u/1 -> Demux/1
  Mux/1 -> y/1

== system Satellite_Model_new_seperateSA/Flexible appendage SA2/6x6 v-u_rotation3 ==
  u : Inport  PortDimensions=6
  Demux : Demux  Outputs=[3 3]
  Mux : Mux  Inputs=[3 3]
  Subsystem : Subsystem
  Subsystem1 : Subsystem
  y : Outport  VectorParamsAs1DForOutWhenUnconnected=off
  wires:
  Subsystem1/1(Out1) -> Mux/2
  Subsystem/1(Out1) -> Mux/1
  Demux/2 -> Subsystem1/1(In1)
  Demux/1 -> Subsystem/1(In1)
  u/1 -> Demux/1
  Mux/1 -> y/1

== system Satellite_Model_new_seperateSA/Flexible appendage SA2/Solar Array 2 ==
  Xddot,P : Inport  PortDimensions=6
  Demux : Demux  Outputs=[6]
  Gain : RCTblocks/Uncertain State Space  Tag=USS  USystem=Mdyn  UValue=[]  X0=[]  uX0=[]
  Mux : Mux  Inputs=[6]
  W_body/.,P : Outport
  wires:
  Mux/1 -> Gain/1
  Gain/1 -> Demux/1
  Xddot,P/1 -> Mux/1
  Demux/1 -> W_body/.,P/1

== system Satellite_Model_new_seperateSA/Instrument /Multi port rigid body ==
  Xddot,P1 : Inport  PortDimensions=6
  Demux : Demux  Outputs=[6]
  Gain : RCTblocks/Uncertain State Space  Tag=USS  USystem=uss(InvDyn)  UValue=[]  X0=[]  uX0=[]
  Mux : Mux  Inputs=[6]
  W_body/.,P1 : Outport
  wires:
  Demux/1 -> W_body/.,P1/1
  Xddot,P1/1 -> Mux/1
  Gain/1 -> Demux/1
  Mux/1 -> Gain/1

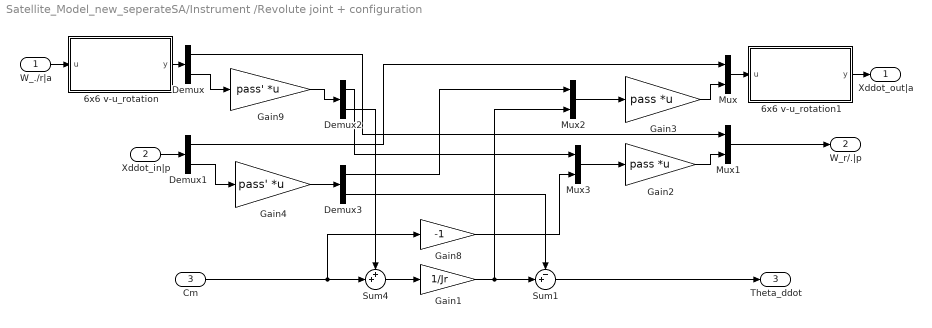
== system Satellite_Model_new_seperateSA/Instrument /Revolute joint + configuration ==
  W_./r|a : Inport  PortDimensions=6
  Xddot_in|p : Inport  Port=2  PortDimensions=6
  Cm : Inport  Port=3  PortDimensions=1
  6x6 v-u_rotation : Subsystem  mask(6x6 rotation matrix (around a given axis)){ra=ra, theta=theta, transp=off}
      mask prompts: ra "Rotation axis (3x1 vector)"; theta "Angle (rad)"; transp "Matrix transposed"
      mask help:
      | For 6 d.o.f. body motion (3 translations and 3 rotations), this block Implement the 6x6 rotation matrix (or its transposed) for a given angle around a given axis.
      |
      | Angle  (rad) can be an uncertain parameter declared with "ureal" with mode 'Range'
      | Ex: ureal('NAME',0,'Range',[-pi pi])
      | Then, ULINEARIZE will provide a model involving the block named "tan_NAME_div4".
      mask init:
      | vUrotation3x3
      mask Help: web('Doc6vurotation.html')
      mask Display:
      | disp('v-rot\n6x6')
      | if transp
      |     port_label('input', 1, '[.]_R1')
      |     port_label('output', 1, '[.]_R2')
      | else
      |     port_label('input', 1, '[.]_R2')
      |     port_label('output', 1, '[.]_R1')
      | end
  6x6 v-u_rotation1 : Subsystem  mask(6x6 rotation matrix (around a given axis)){ra=ra, theta=theta, transp=on}
      mask prompts: ra "Rotation axis (3x1 vector)"; theta "Angle (rad)"; transp "Matrix transposed"
      mask help:
      | For 6 d.o.f. body motion (3 translations and 3 rotations), this block Implement the 6x6 rotation matrix (or its transposed) for a given angle around a given axis.
      |
      | Angle  (rad) can be an uncertain parameter declared with "ureal" with mode 'Range'
      | Ex: ureal('NAME',0,'Range',[-pi pi])
      | Then, ULINEARIZE will provide a model involving the block named "tan_NAME_div4".
      mask init:
      | vUrotation3x3
      mask Help: web('Doc6vurotation.html')
      mask Display:
      | disp('v-rot\n6x6')
      | if transp
      |     port_label('input', 1, '[.]_R1')
      |     port_label('output', 1, '[.]_R2')
      | else
      |     port_label('input', 1, '[.]_R2')
      |     port_label('output', 1, '[.]_R1')
      | end
  Demux : Demux  Outputs=[3 3]
  Demux1 : Demux  Outputs=[3 3]
  Demux2 : Demux  Outputs=[2 1]
  Demux3 : Demux  Outputs=[2 1]
  Gain1 : Gain  Gain=1/Jr
  Gain2 : Gain  Gain=pass  Multiplication=Matrix(K*u) (u vector)
  Gain3 : Gain  Gain=pass  Multiplication=Matrix(K*u) (u vector)
  Gain4 : Gain  Gain=pass'  Multiplication=Matrix(K*u) (u vector)
  Gain8 : Gain  Gain=-1
  Gain9 : Gain  Gain=pass'  Multiplication=Matrix(K*u) (u vector)
  Mux : Mux  Inputs=[3 3]
  Mux1 : Mux  Inputs=[3 3]
  Mux2 : Mux  Inputs=[2 1]
  Mux3 : Mux  Inputs=[2 1]
  Sum1 : Sum  Inputs=-+|
  Sum4 : Sum  Inputs=++|
  Xddot_out|a : Outport  VectorParamsAs1DForOutWhenUnconnected=off
  W_r/.|p : Outport  Port=2  VectorParamsAs1DForOutWhenUnconnected=off
  Theta_ddot : Outport  Port=3  VectorParamsAs1DForOutWhenUnconnected=off
  wires:
  W_./r|a/1 -> 6x6 v-u_rotation/1(u)
  Mux1/1 -> W_r/.|p/1
  Demux1/1 -> Mux/1
  Cm/1 -> Gain8/1, Sum4/2
  Demux/1 -> Mux1/1
  Gain2/1 -> Mux1/2
  Sum1/1 -> Theta_ddot/1
  Demux/2 -> Gain9/1
  Gain1/1 -> Mux2/2, Sum1/2
  Xddot_in|p/1 -> Demux1/1
  Sum4/1 -> Gain1/1
  Gain3/1 -> Mux/2
  Demux3/2 -> Sum1/1
  Gain9/1 -> Demux2/1
  Demux2/2 -> Sum4/1
  Mux2/1 -> Gain3/1
  Demux1/2 -> Gain4/1
  Gain4/1 -> Demux3/1
  Mux3/1 -> Gain2/1
  Gain8/1 -> Mux3/2
  Demux2/1 -> Mux3/1
  Demux3/1 -> Mux2/1
  6x6 v-u_rotation/1(y) -> Demux/1
  6x6 v-u_rotation1/1(y) -> Xddot_out|a/1
  Mux/1 -> 6x6 v-u_rotation1/1(u)

== system Satellite_Model_new_seperateSA/Multi port rigid body + revolute joint/Multi port rigid body ==
  Xddot,P1 : Inport  PortDimensions=6
  W_./body,P2 : Inport  Port=2  PortDimensions=6
  Demux : Demux  Outputs=[6 6]
  Gain : RCTblocks/Uncertain State Space  Tag=USS  USystem=uss(InvDyn)  UValue=[]  X0=[]  uX0=[]
  Mux : Mux  Inputs=[6 6]
  W_body/.,P1 : Outport
  Xddot,P2 : Outport  Port=2
  wires:
  Mux/1 -> Gain/1
  Gain/1 -> Demux/1
  Xddot,P1/1 -> Mux/1
  Demux/1 -> W_body/.,P1/1
  W_./body,P2/1 -> Mux/2
  Demux/2 -> Xddot,P2/1
